simulink model "PID_FIS_Controller"  (R2020b)
settings: Solver=VariableStepAuto  StartTime=0.0  StopTime=20  RelTol=1e-3
libraries: fuzblock x1, simulink x1
settings Model: Creator=smsmt  LastModifiedBy=smsmt

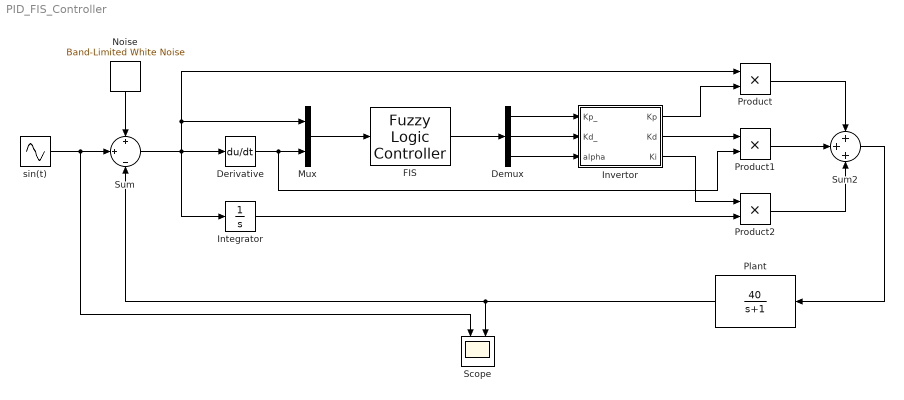
== system PID_FIS_Controller ==
  Demux : Demux  Outputs=3
  Derivative : Derivative
  FIS : fuzblock/Fuzzy Logic  Controller  FIS=PID_FIS  OutputSampleNumber=101  DataType=double  FuzzifiedInputs=off  RuleFiringStrengths=off  RuleOutputs=off  AggregatedOutputs=off  SimulateUsing=Interpreted execution  OutOfRangeInputValueMessage=warning  NoRuleFiredMessage=warning  EmptyOutputFuzzySetMessage=warning
  Integrator : Integrator
  Invertor : MATLAB Function  TreatAsAtomicUnit=on
  Mux : Mux  Inputs=2
  Noise : simulink/Sources/Band-Limited White Noise  Cov=[0.001]  Ts=0.1  seed=[23341]
  Plant : TransferFcn  Numerator=[40]  Denominator=[1 1]
  Product : Product
  Product1 : Product
  Product2 : Product
  Scope : Scope  NumInputPorts=2
  Sum : Sum  Inputs=+|+|-
  Sum2 : Sum  Inputs=+++
  sin(t) : Sin  SampleTime=0
  wires:
  FIS/1 -> Demux/1
  Mux/1 -> FIS/1
  Derivative/1 -> Mux/2, Product1/2
  Sum/1 -> Derivative/1, Mux/1, Product/1, Integrator/1
  Demux/1 -> Invertor/1(Kp_)
  Demux/2 -> Invertor/2(Kd_)
  Demux/3 -> Invertor/3(alpha)
  Plant/1 -> Sum/3, Scope/2
  sin(t)/1 -> Sum/2, Scope/1
  Product/1 -> Sum2/1
  Product2/1 -> Sum2/3
  Invertor/1(Kp) -> Product/2
  Invertor/2(Kd) -> Product1/1
  Invertor/3(Ki) -> Product2/1
  Integrator/1 -> Product2/2
  Noise/1 -> Sum/1
  Product1/1 -> Sum2/2
  Sum2/1 -> Plant/1

== matlab function PID_FIS_Controller/Invertor ==
  data: Kp output; Kd output; Kp_ input; Kd_ input; alpha input; Ki output
function [Kp, Kd, Ki]= fcn(Kp_, Kd_, alpha)
    Kp_min = 0;
    Kp_max = 0.06;
    Kd_min = 0;
    Kd_max = 0.01;
    Kp = (Kp_max - Kp_min) * Kp_ + Kp_min;
    Kd = (Kd_max - Kd_min) * Kd_ + Kd_min;
    Ki = (Kp ^ 2) / (alpha * Kd);
